simulink model "wang_jingyang_0900085786"  (R2022a)
settings: Solver=FixedStepAuto  StartTime=0.0  StopTime=1  FixedStep=1e-06  MaxStep=1e-6  RelTol=1e-3
values from neighbouring files (symbols this model uses):
  fsw = 1000000    [wang_jingyang_0900085786_parameter.m]
  J = 183e-07    (= 1.83e-05)    [wang_jingyang_0900085786_parameter.m]
  kt = 0.137    [wang_jingyang_0900085786_parameter.m]
  max_current = 2.8    [wang_jingyang_0900085786_parameter.m]
  period_duty = 1    [wang_jingyang_0900085786_parameter.m]
  r = 6.61    [wang_jingyang_0900085786_parameter.m]
  rs = 0.72    [wang_jingyang_0900085786_parameter.m]
  torque_slope = 2.646E-04    (= 0.0002646)    [wang_jingyang_0900085786_parameter.m]
  vs = 72    [wang_jingyang_0900085786_parameter.m]
libraries: nesl_utility x13, ee_lib x10, fl_lib x9, spsMeanLib x2, simulink x2
settings Model: Creator=claudio.rossi  LastModifiedBy=JasonIrayshon
settings SolverCC: ZeroCrossAlgorithm=Adaptive
settings DataIOCC: SaveFormat=Array
settings DebuggingCC: IgnoredZcDiagnostic=none  UnconnectedInputMsg=warning  UnconnectedOutputMsg=warning  UnconnectedLineMsg=warning
settings RTWCC: DLArmComputeVersion=19.05

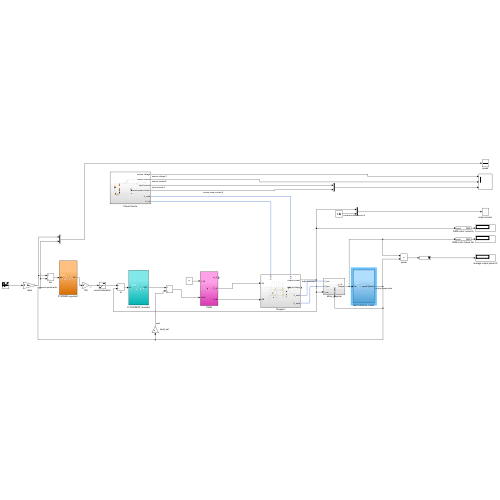
[thumbnail: Simulink's stored preview of the top-level diagram]
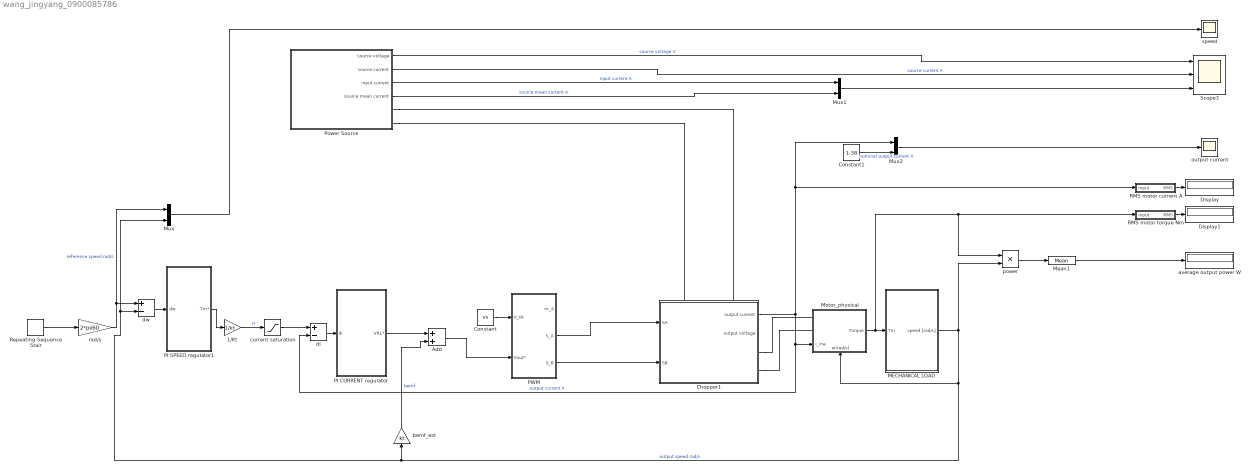
== system wang_jingyang_0900085786 ==
  1/Kt : Gain  Gain=1/kt
  Add : Sum
  Chopper1 : Subsystem
      settings: PortSchema="{\"entries\":[{\"content\":{\"sides\":[{\"content\":{\"connectorIds\":[\"In1\",\"In2\"]},\"type\":\"ConnectorPlacement.EquallySpacedRectSide\",\"uuid\":\"6b8cc3de-865d-4570-879b-f9024d4fd7e5\"},{\"content\":{\"connectorIds\":[\"Out1\",\"Out2\",\"RConn1\",\"RConn2\"],\"side\":\"RIGHT\"},\"type\":\"ConnectorPlacement.EquallySpacedRectSide\",\"uuid\":\"7f03e7c5-24a6-417f-989e-25a3d60ab139\"},{\"content\":{\"connectorIds\":[\"LConn1\",\"LConn2\"],\"side\":\"TOP\"},\"type\":\"ConnectorPlacement.EquallySpacedRectSide\",\"uuid\":\"d8aa3f33-fa7f-4dd9-94c6-a8d4ddf046a0\"},{\"content\":{\"connectorIds\":[],\"side\":\"BOTTOM\"},\"type\":\"ConnectorPlacement.EquallySpacedRectSide\",\"uuid\":\"82a3c5ca-95ba-41a9-9ebb-951a0a94f788\"}]},\"type\":\"ConnectorPlacement.EquallySpacedConnector\",\"uuid\":\"1a04d642-2b5e-450e-b011-8676eb2fa378\"}],\"packageUris\":[\"http://schema.mathworks.com/mf0/Connector/R2020b\"],\"version\":\"1.0\"}"
  Constant : Constant  Value=vs
  Constant1 : Constant  Value=1.38
  Display : Display
  Display1 : Display
  MECHANICAL LOAD : Subsystem
  Mean1 : spsMeanLib/Mean  Freq=fsw  Vinit=0  Ts=0
  Motor_physical : Subsystem
      settings: PortSchema="{\"entries\":[{\"content\":{\"sides\":[{\"content\":{\"connectorIds\":[\"LConn1\",\"LConn2\",\"In1\"]},\"type\":\"ConnectorPlacement.EquallySpacedRectSide\",\"uuid\":\"b6037c4a-1f3a-465c-bacb-bde747a26b4c\"},{\"content\":{\"connectorIds\":[\"Out1\"],\"side\":\"RIGHT\"},\"type\":\"ConnectorPlacement.EquallySpacedRectSide\",\"uuid\":\"519ff893-bc94-47bb-a520-d8eddd14445d\"},{\"content\":{\"connectorIds\":[],\"side\":\"TOP\"},\"type\":\"ConnectorPlacement.EquallySpacedRectSide\",\"uuid\":\"9e95d8c6-7747-4ab4-a157-2e1e9a78c15e\"},{\"content\":{\"connectorIds\":[\"In2\"],\"side\":\"BOTTOM\"},\"type\":\"ConnectorPlacement.EquallySpacedRectSide\",\"uuid\":\"be1431e5-ccb9-4c79-a3a9-fcb6f60af3f0\"}]},\"type\":\"ConnectorPlacement.EquallySpacedConnector\",\"uuid\":\"2d312488-f543-490d-bb4c-a0f0f3bfbb5e\"}],\"packageUris\":[\"http://schema.mathworks.com/mf0/Connector/R2020b\"],\"version\":\"1.0\"}"
  Mux : Mux  Inputs=2
  Mux1 : Mux  Inputs=2
  Mux2 : Mux  Inputs=2
  PI CURRENT regulator : Subsystem
  PI SPEED regulator1 : Subsystem
  PWM : Subsystem
  Power Source : Subsystem
  RMS motor current A : Subsystem  mask{t=period_duty}
      mask prompts: t "Integrating time T [s]"
      mask DialogControl DescTextVar Prompt: Mean value calculator over period T
  RMS motor torque Nm : Subsystem  mask{t=period_duty}
      mask prompts: t "Integrating time T [s]"
      mask DialogControl DescTextVar Prompt: Mean value calculator over period T
  Repeating Sequence Stair : simulink/Sources/Repeating Sequence Stair  OutValues="[0 3375 3375  -1350 675 675 1350 1350 3375 3375].'"  tsamp=0.1  OutMin=[]  OutMax=[]  OutDataTypeStr=double  OutputDataTypeScalingMode=double  OutDataType=fixdt(0,8)  ConRadixGroup=Best Precision: Vector-wise  OutScaling=2^-12
  Scope3 : Scope  NumInputPorts=3
  average output power W : Display
  bemf_est : Gain  Gain=kt
  current saturation : Saturate  UpperLimit=max_current/2  LowerLimit=-max_current/2
  di : Sum  Inputs=+-
  dw : Sum  Inputs=+-
  "output current " : Scope
  power : Product
  rad/s : Gain  Gain=2*pi/60
  speed : Scope
  wires:
  di/1 -> PI CURRENT regulator/1(di)
  bemf_est/1 -> Add/2  "bemf"
  MECHANICAL LOAD/1(speed [rad/s]) -> power/2, Mux/2, dw/2, bemf_est/1, Motor_physical/2(w(rad/s))  "output speed rad/s"
  PI SPEED regulator1/1(Tm*) -> 1/Kt/1
  rad/s/1 -> Mux/1, dw/1  "reference speed rad/s"
  dw/1 -> PI SPEED regulator1/1(dw)
  current saturation/1 -> di/1
  1/Kt/1 -> current saturation/1  "I*"
  RMS motor current A/1(RMS) -> Display/1
  Mux/1 -> speed/1
  PI CURRENT regulator/1(VRL*) -> Add/1
  PWM/2(S_A) -> Chopper1/1(SA)
  PWM/3(S_B) -> Chopper1/2(SB)
  Add/1 -> PWM/2(Vout*)
  RMS motor torque Nm/1(RMS) -> Display1/1
  Chopper1/1(output current) -> RMS motor current A/1(input), Mux2/1, di/2, Motor_physical/1(I_ina)  "output current A"
  Motor_physical/1(Torque) -> RMS motor torque Nm/1(input), power/1, MECHANICAL LOAD/1(Tm)
  Constant/1 -> PWM/1(V_IN)
  Repeating Sequence Stair/1 -> rad/s/1
  Power Source/1(source voltage) -> Scope3/1  "source voltage V"
  Power Source/2(source current) -> Scope3/2  "source current A"
  Power Source/4("source mean current ") -> Mux1/2  "source mean current A"
  Power Source/3(input current) -> Mux1/1  "input current A"
  Mux1/1 -> Scope3/3
  Constant1/1 -> Mux2/2  "nominal output current A"
  Mux2/1 -> "output current "/1
  power/1 -> Mean1/1
  Mean1/1 -> average output power W/1
  connections:
  Power Source/RConn1 -- Chopper1/LConn2
  Power Source/RConn2 -- Chopper1/LConn1
  Chopper1/RConn1 -- Motor_physical/LConn1
  Chopper1/RConn2 -- Motor_physical/LConn2

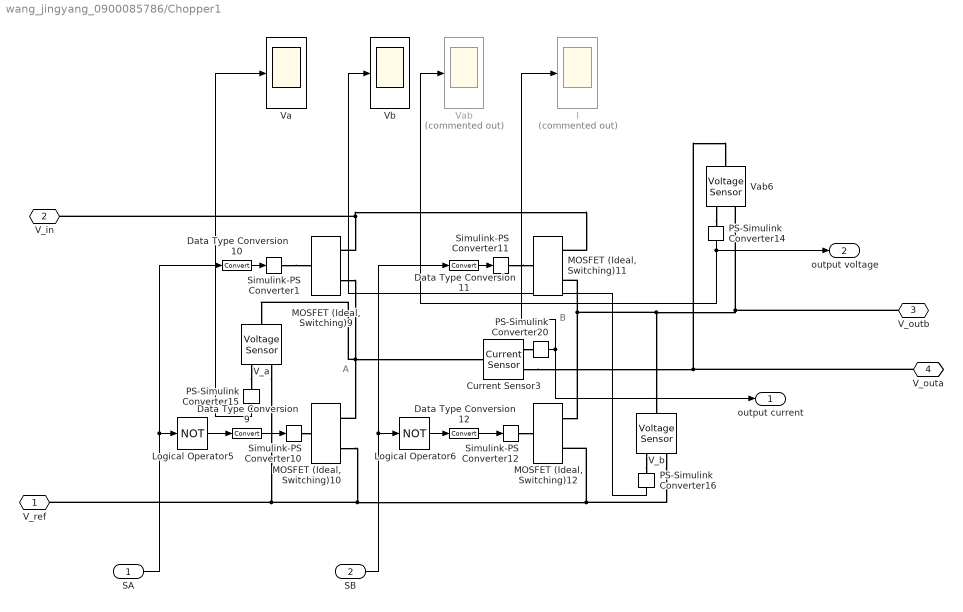
== system wang_jingyang_0900085786/Chopper1 ==
  note: A
  note: B
  SA : Inport
  SB : Inport  Port=2
  Current Sensor3 : fl_lib/Electrical/Electrical Sensors/Current Sensor
      settings: SourceProductBaseCode=PW,SS,VE
  Data Type Conversion{9..12} (4 alike) : DataTypeConversion  SaturateOnIntegerOverflow=off  RndMeth=Floor
  I : Scope  Commented=on
  Logical Operator5 : Logic  Operator=NOT  AllPortsSameDT=off  OutDataTypeStr=boolean
  Logical Operator6 : Logic  Operator=NOT  AllPortsSameDT=off  OutDataTypeStr=boolean
  MOSFET (Ideal, Switching){9..12} (4 alike) : ee_lib/Semiconductors & Converters/MOSFET (Ideal, Switching)  Rds=0.01 Ohm  Goff=1e-6 1/Ohm  Vth=0.5 V  diode_param=1  diode_Vf=0.8 V  diode_Ron=0.001 Ohm  diode_Goff=1e-5 1/Ohm  diode_C=50e-9 F  diode_iRM=-235 A  diode_iF=300 A  diode_idot=-50 A/us  diode_trr_param=1  diode_trr_factor=3  diode_trr=15 us  diode_Qrr=1500 s*uA  thermal_loss_option=ee.enum.converters.thermalLossOption.constantvalues  Von_data=[0, 1.1, 1.3, 1.45, 1.75, 2.25, 2.7; 0, 1, 1.15, 1.35, 1.7, 2.35, 3] V  Tj=[298.15, 398.15] K  Iout_data=[0, 10, 50, 100, 200, 400, 600] A  Eon_data=[0, .29, 1.43, 2.86, 5.71, 13.14, 22.86; 0, .57, 2.63, 5.14, 10.29, 20.57, 30.29] * 1e-3 J  Eoff_data=[0, .21, 1.07, 2.14, 4.29, 9.86, 17.14; 0, .43, 1.97, 3.86, 7.71, 15.43, 22.71] * 1e-3 J  Tj_loss=[298.15, 398.15] K  Iout_data_loss=[0, 10, 50, 100, 200, 400, 600] A  Eon_scalar=22.86e-3 J  Eoff_scalar=17.14e-3 J  Voff=300 V  Iout_scalar=600 A  diodeModelType=ee.enum.converters.diodeModelType.pwl  diodeTableType=ee.enum.diode.tableType.IfMat  diode_IfMat=[.07, .12, .19, 1.75, 4.24, 7.32, 11.2; .16, .3, .72, 2.14, 4.02, 6.35, 9.12] A  diode_VfMat=[.9, 1.15, 1.25, 1.5, 1.75, 2.17, 2.6, 2.85; .58, .68, .75, 1.1, 1.38, 1.77, 2.27, 2.7] V  diode_TjVec=[25, 125] degC  diode_VfVec=[.5, .7, .9, 1.3, 1.7, 2.1, 2.5] V  diode_IfVec=[.1, .2, .5, 1, 2, 4, 7, 10] A  diode_Vr=-600 V  diode_Ls=150 nH  diode_Erec=0.03 J  thermal_network_parameterization=ee.enum.thermalNetworkTopology.external  Rth=[.03, .2] K/W  Rth_Cauer=[.03, .1, .2] K/W  Rth_Foster=[.03, .2] K/W  thermal_mass_parameterization=ee.enum.thermalNetwork.timeconstant  thermal_mass=[3, 25] J/K  thermal_mass_Cauer=[3, 10, 25] J/K  thermal_mass_Foster=[33, 50] J/K  thermal_time_constant=[.1, 5] s  thermal_time_constant_Cauer=[.1, 1, 5] s  thermal_time_constant_Foster=[1, 10] s  thermal_mass_initial_temperatures=[25, 25] degC  thermal_mass_initial_temperatures_Cauer=[25, 25, 25] degC  junction_thermal_mass=0.1 J/K  steadyState_Foster=simscape.enum.onoff.on  Tvec_initial_Foster=[25, 25, 25, 25] degC  no_thermal_network=0  junction_temperature_specify=off  junction_temperature_priority=None  junction_temperature=25 degC  junction_temperature_nominal_specify=off  junction_temperature_nominal_unit=degC  junction_temperature_nominal_value=1  vT_specify=off  vT_priority=None  vT=0 V  vT_nominal_specify=off  vT_nominal_unit=V  vT_nominal_value=1  Qj_specify=off  Qj_priority=None  Qj=0 W  Qj_nominal_specify=off  Qj_nominal_unit=W  Qj_nominal_value=1
  PS-Simulink Converter{14..16,20} (4 alike) : nesl_utility/PS-Simulink Converter  PhysicalDomain=network_engine_domain  SubClassName=ps_output  LeftPortType=input  RightPortType=output  PseudoPeriodic=off  Frequencies=[]  VectorFormat=inherit  Unit=inherit  AffineConversion=off
      settings: SourceProductBaseCode=SS,PW,VE
  Simulink-PS Converter{1,10..12} (4 alike) : nesl_utility/Simulink-PS Converter  PhysicalDomain=network_engine_domain  SubClassName=ps_input  LeftPortType=input  RightPortType=output  PseudoPeriodic=off  Frequencies=[]  NoiseDistribution=none  NoiseParameters=[]  Unit=1  AffineConversion=off  FilteringAndDerivatives=provide  SimscapeFilterOrder=1  InputFilterTimeConstant=0.001  UdotUserProvided=0
      settings: SourceProductBaseCode=SS,PW,VE
  V_a : fl_lib/Electrical/Electrical Sensors/Voltage Sensor
      settings: SourceProductBaseCode=PW,SS,VE
  V_b : fl_lib/Electrical/Electrical Sensors/Voltage Sensor
      settings: SourceProductBaseCode=PW,SS,VE
  Va : Scope
  Vab : Scope  Commented=on
  Vab6 : fl_lib/Electrical/Electrical Sensors/Voltage Sensor
      settings: SourceProductBaseCode=PW,SS,VE
  Vb : Scope
  V_ref : PMIOPort  Side=Left
  V_in : PMIOPort  Port=2  Side=Left
  V_outb : PMIOPort  Port=3  Side=Right
  V_outa : PMIOPort  Port=4  Side=Right
  output current : Outport
  output voltage : Outport  Port=2
  wires:
  Data Type Conversion9/1 -> Simulink-PS Converter10/1
  Logical Operator5/1 -> Data Type Conversion9/1
  SA/1 -> Data Type Conversion10/1, Logical Operator5/1
  PS-Simulink Converter15/1 -> Va/1
  Data Type Conversion11/1 -> Simulink-PS Converter11/1
  PS-Simulink Converter16/1 -> Vb/1
  Data Type Conversion12/1 -> Simulink-PS Converter12/1
  Logical Operator6/1 -> Data Type Conversion12/1
  Data Type Conversion10/1 -> Simulink-PS Converter1/1
  PS-Simulink Converter20/1 -> I/1, output current/1
  PS-Simulink Converter14/1 -> output voltage/1, Vab/1
  SB/1 -> Logical Operator6/1, Data Type Conversion11/1
  connections:
  V_a/RConn1 -- PS-Simulink Converter15/LConn1
  "MOSFET (Ideal, Switching)12"/RConn2 -- "MOSFET (Ideal, Switching)10"/RConn2 -- V_ref/RConn1 -- V_a/RConn2 -- V_b/RConn2
  Current Sensor3/RConn2 -- Vab6/LConn1 -- V_outa/RConn1
  Simulink-PS Converter1/RConn1 -- "MOSFET (Ideal, Switching)9"/LConn1
  V_b/LConn1 -- V_outb/RConn1 -- Vab6/RConn2 -- "MOSFET (Ideal, Switching)11"/RConn2 -- "MOSFET (Ideal, Switching)12"/RConn1
  Current Sensor3/RConn1 -- PS-Simulink Converter20/LConn1
  "MOSFET (Ideal, Switching)10"/RConn1 -- V_a/LConn1 -- Current Sensor3/LConn1 -- "MOSFET (Ideal, Switching)9"/RConn2
  "MOSFET (Ideal, Switching)11"/RConn1 -- V_in/RConn1 -- "MOSFET (Ideal, Switching)9"/RConn1
  Vab6/RConn1 -- PS-Simulink Converter14/LConn1
  Simulink-PS Converter12/RConn1 -- "MOSFET (Ideal, Switching)12"/LConn1
  Simulink-PS Converter10/RConn1 -- "MOSFET (Ideal, Switching)10"/LConn1
  Simulink-PS Converter11/RConn1 -- "MOSFET (Ideal, Switching)11"/LConn1
  V_b/RConn1 -- PS-Simulink Converter16/LConn1

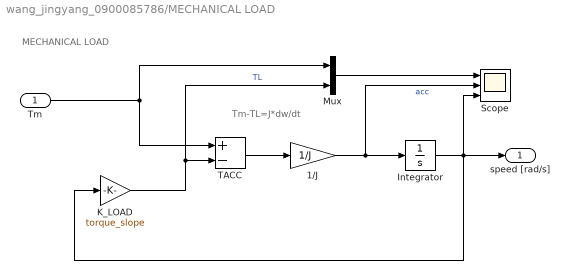
== system wang_jingyang_0900085786/MECHANICAL LOAD ==
  note: MECHANICAL LOAD
  note: Tm-TL=J*dw/dt
  Tm : Inport
  1/J : Gain  Gain=1/J
  Integrator : Integrator
  K_LOAD : Gain  Gain=torque_slope
  Mux : Mux  Inputs=2
  Scope : Scope  NumInputPorts=3
  TACC : Sum  Inputs=+-
  speed [rad/s] : Outport
  wires:
  Tm/1 -> Mux/1, TACC/1
  K_LOAD/1 -> Mux/2, TACC/2  "TL"
  TACC/1 -> 1/J/1
  1/J/1 -> Scope/2, Integrator/1  "acc"
  Integrator/1 -> Scope/3, K_LOAD/1, speed [rad/s]/1
  Mux/1 -> Scope/1

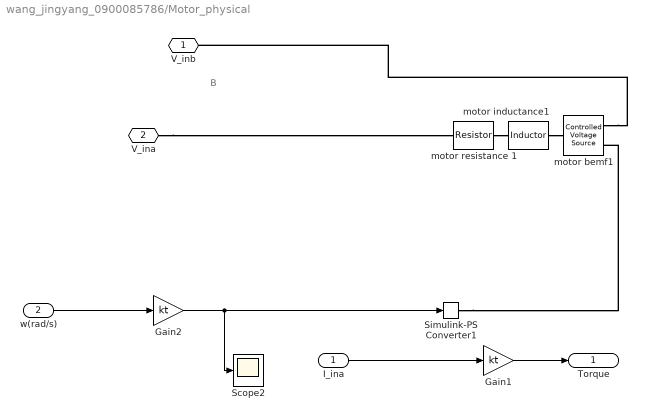
== system wang_jingyang_0900085786/Motor_physical ==
  note: B
  I_ina : Inport
  w(rad/s) : Inport  Port=2
  Gain1 : Gain  Gain=kt
  Gain2 : Gain  Gain=kt
  Scope2 : Scope
  Simulink-PS Converter1 : nesl_utility/Simulink-PS Converter  PhysicalDomain=network_engine_domain  SubClassName=ps_input  LeftPortType=input  RightPortType=output  PseudoPeriodic=off  Frequencies=[]  NoiseDistribution=none  NoiseParameters=[]  Unit=1  AffineConversion=off  FilteringAndDerivatives=provide  SimscapeFilterOrder=1  InputFilterTimeConstant=0.001  UdotUserProvided=0
      settings: SourceProductBaseCode=SS,PW,VE
  motor inductance1 : ee_lib/Passive/Inductor  l=l H  enable_L_tol=0  L_tol=20  tol_distribution=1  nSigma=4  r=0 Ohm  g=1e-9 1/Ohm  enable_operating_limits=0  operating_limit_action=2  max_working_current=1 A  power_rating=1 W  enable_faults=0  fault_action=1  lambdaPercent=50  k_faulted=0.9999  turnsShort=0  openCct=0  groundShort=0  groundShortG=0 1/Ohm  tau_fault=1e-3 s  enable_temporal_fault=0  t_fault=1 s  enable_behavioral_fault=0  max_permissible_voltage=100 V  n_fail_on_voltage=1  max_permissible_current=1 A  t_fail_on_current=1 s  i_L_specify=off  i_L_priority=High  i_L=0 A  i_L_nominal_specify=off  i_L_nominal_unit=A  i_L_nominal_value=1
  motor resistance 1 : ee_lib/Passive/Resistor  R=r Ohm  enable_R_tol=0  R_tol=5  tol_distribution=1  nSigma=4  enable_operating_limits=0  operating_limit_action=2  max_working_voltage=100 V  power_rating=1 W  enable_faults=0  fault_action=1  R_faulted=inf Ohm  enable_temporal_fault=0  t_fault=1 s  enable_behavioral_fault=0  max_permissible_current=1 A  t_fail_on_current=1 s  noise_mode=0  sample_time=1e-3 s  repeatability=1  auto_seed=4144164703  user_seed=0  Tdevice=25 degC  power_derating_T1=70 degC  power_derating_T2=155 degC  operating_temperature_range_vec=[-50, 150] degC  alpha=3.93e-3 1/K  Tmeas=25 degC  thermal_mass=100 J/K  temperature_specify=off  temperature_priority=High  temperature=298.15 K  temperature_nominal_specify=off  temperature_nominal_unit=K  temperature_nominal_value=1
  motor bemf1 : fl_lib/Electrical/Electrical Sources/Controlled Voltage Source
      settings: SourceProductBaseCode=PW,SS,VE
  V_inb : PMIOPort  Side=Left
  V_ina : PMIOPort  Port=2  Side=Left
  Torque : Outport
  wires:
  I_ina/1 -> Gain1/1
  Gain2/1 -> Scope2/1, Simulink-PS Converter1/1
  Gain1/1 -> Torque/1
  w(rad/s)/1 -> Gain2/1
  connections:
  motor resistance 1/RConn1 -- motor inductance1/LConn1
  motor bemf1/RConn2 -- V_inb/RConn1
  V_ina/RConn1 -- motor resistance 1/LConn1
  Simulink-PS Converter1/RConn1 -- motor bemf1/RConn1
  motor inductance1/RConn1 -- motor bemf1/LConn1

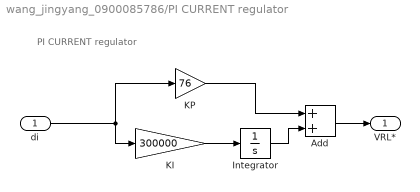
== system wang_jingyang_0900085786/PI CURRENT regulator ==
  note: PI CURRENT regulator
  di : Inport
  Add : Sum
  Integrator : Integrator
  KI : Gain  Gain=300000
  KP : Gain  Gain=76
  VRL* : Outport
  wires:
  Integrator/1 -> Add/2
  di/1 -> KP/1, KI/1
  KP/1 -> Add/1
  KI/1 -> Integrator/1
  Add/1 -> VRL*/1

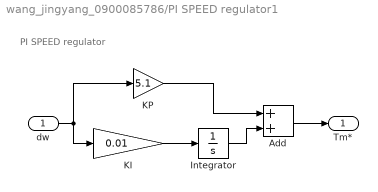
== system wang_jingyang_0900085786/PI SPEED regulator1 ==
  note: PI SPEED regulator
  dw : Inport
  Add : Sum
  Integrator : Integrator
  KI : Gain  Gain=0.01
  KP : Gain  Gain=5.1
  Tm* : Outport
  wires:
  Add/1 -> Tm*/1
  KI/1 -> Integrator/1
  KP/1 -> Add/1
  dw/1 -> KI/1, KP/1
  Integrator/1 -> Add/2

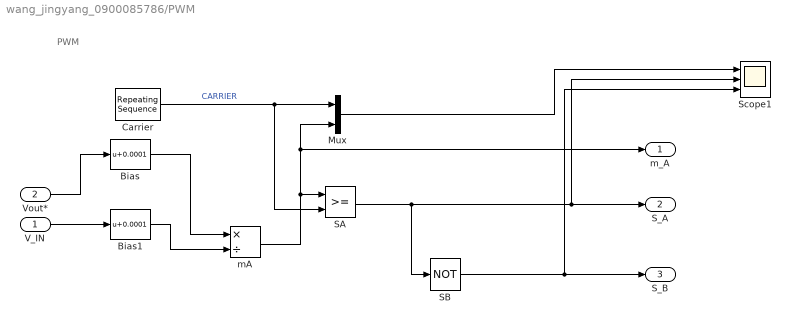
== system wang_jingyang_0900085786/PWM ==
  note: PWM
  V_IN : Inport
  Vout* : Inport  Port=2
  Bias : Bias  Bias=0.0001  SaturateOnIntegerOverflow=off
  Bias1 : Bias  Bias=0.0001  SaturateOnIntegerOverflow=off
  Carrier : simulink/Sources/Repeating Sequence  rep_seq_t="[0 1/fsw/2  1/fsw]"  rep_seq_y=[-1 1 -1]
  Mux : Mux  Inputs=2
  SA : RelationalOperator  OutDataTypeStr=boolean  RndMeth=Simplest  InputSameDT=off
  SB : Logic  Operator=NOT  AllPortsSameDT=off  OutDataTypeStr=boolean
  Scope1 : Scope  NumInputPorts=3
  mA : Product  Inputs=*/
  m_A : Outport
  S_A : Outport  Port=2
  S_B : Outport  Port=3
  wires:
  Carrier/1 -> SA/2, Mux/1  "CARRIER"
  SA/1 -> SB/1, Scope1/2, S_A/1
  Mux/1 -> Scope1/1
  mA/1 -> Mux/2, m_A/1, SA/1
  SB/1 -> Scope1/3, S_B/1
  Vout*/1 -> Bias/1
  Bias/1 -> mA/1
  V_IN/1 -> Bias1/1
  Bias1/1 -> mA/2

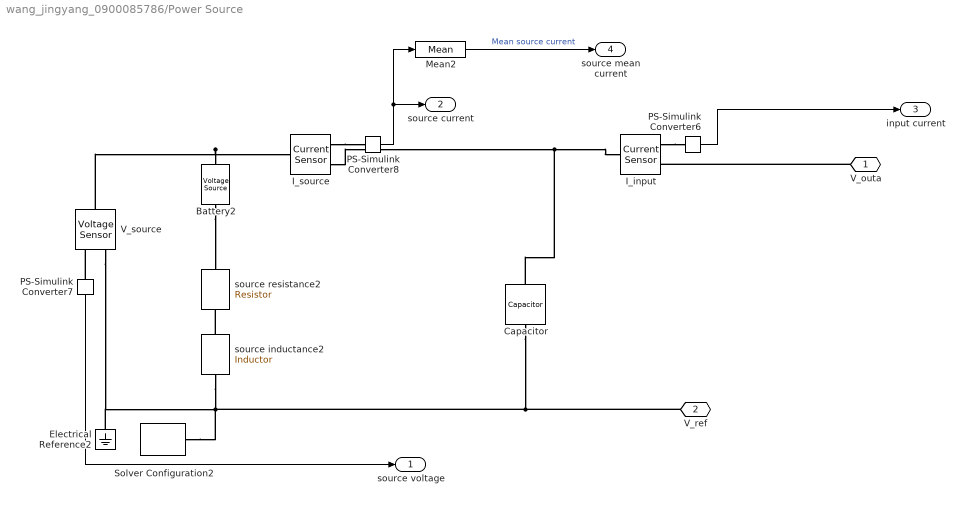
== system wang_jingyang_0900085786/Power Source ==
  Battery2 : ee_lib/Sources/Voltage Source  dc_voltage=vs V  ac_voltage=0 V  ac_shift=0 rad  ac_frequency=60 Hz  noise_mode=0  PSD=0 V^2/Hz  repeatability=1  auto_seed=676943032  user_seed=0  sample_time=1e-3 s  i_specify=off  i_priority=None  i=0 A  i_nominal_specify=off  i_nominal_unit=A  i_nominal_value=1  v_specify=off  v_priority=None  v=0 V  v_nominal_specify=off  v_nominal_unit=V  v_nominal_value=1
  Capacitor : ee_lib/Passive/Capacitor  cap_option=0  c=940e-5 F  Cvec=[1e-05, 1e-06] F  Vvec=[0, 10] V  CV_table_symmetry=1  f_vec=[1, 10] kHz  DFext_vec=[.8, 1.2]  enable_C_tol=0  C_tol=5  tol_distribution=1  nSigma=4  r=0.21 Ohm  g=0 1/Ohm  averaging_period=0 s  enable_operating_limits=0  operating_limit_action=2  max_working_voltage_range=[-25, 25] V  power_rating=1 W  enable_faults=0  fault_action=1  Cscale_faulted=100  R_faulted=1e-3 Ohm  G_faulted=0 1/Ohm  tau_fault=1e-3 s  enable_temporal_fault=0  t_fault=1 s  enable_behavioral_fault=0  max_permissible_voltage_range=[-100, 100] V  t_fail_on_voltage=1 s  i_specify=off  i_priority=None  i=0 A  i_nominal_specify=off  i_nominal_unit=A  i_nominal_value=1  v_specify=off  v_priority=None  v=0 V  v_nominal_specify=off  v_nominal_unit=V  v_nominal_value=1  vc_specify=off  vc_priority=High  vc=0 V  vc_nominal_specify=off  vc_nominal_unit=V  vc_nominal_value=1
  Electrical Reference2 : fl_lib/Electrical/Electrical Elements/Electrical Reference
      settings: SourceProductBaseCode=PW,SS,VE
  I_input : fl_lib/Electrical/Electrical Sensors/Current Sensor
      settings: SourceProductBaseCode=PW,SS,VE
  I_source : fl_lib/Electrical/Electrical Sensors/Current Sensor
      settings: SourceProductBaseCode=PW,SS,VE
  Mean2 : spsMeanLib/Mean  Freq=fsw  Vinit=0  Ts=0
  PS-Simulink Converter6 : nesl_utility/PS-Simulink Converter  PhysicalDomain=network_engine_domain  SubClassName=ps_output  LeftPortType=input  RightPortType=output  PseudoPeriodic=off  Frequencies=[]  VectorFormat=inherit  Unit=inherit  AffineConversion=off
      settings: SourceProductBaseCode=SS,PW,VE
  PS-Simulink Converter7 : nesl_utility/PS-Simulink Converter  PhysicalDomain=network_engine_domain  SubClassName=ps_output  LeftPortType=input  RightPortType=output  PseudoPeriodic=off  Frequencies=[]  VectorFormat=inherit  Unit=inherit  AffineConversion=off
      settings: SourceProductBaseCode=SS,PW,VE
  PS-Simulink Converter8 : nesl_utility/PS-Simulink Converter  PhysicalDomain=network_engine_domain  SubClassName=ps_output  LeftPortType=input  RightPortType=output  PseudoPeriodic=off  Frequencies=[]  VectorFormat=1-D array  Unit=inherit  AffineConversion=off
      settings: SourceProductBaseCode=SS,PW,VE
  Solver Configuration2 : nesl_utility/Solver Configuration  PhysicalDomain=network_engine_domain  SubClassName=solver  LeftPortType=input  RightPortType=generic  Tones=[]  Harmonics=[]  SimulateNoise=off  Profile=off  UseLocalSampling=off  EnableSwitchedLinearOptims=on  FrequencyDomain=off  UseCCode=off  RelTol=0.001  AbsTol=1e-06  MinStep=1e-09  ToWorkspace=off  RevertToSquareIcSolve=off  NumHomotopyIterations=100  PhasorMode=off  PhasorModeNumHarmonics=1  IndexReductionMethod=DerivativeReplacement  DoDC=off  ResidualTolerance=1e-09  UseLocalSolver=off  LocalSolverChoice=NE_BACKWARD_EULER_ADVANCER  LocalSolverSampleTime=0.001  DoFixedCost=off  MaxNonlinIter=3  MaxModeIter=2  ComputeImpulses=off  ImpulseIterations=2  LinearAlgebra=auto  LinearAlgebraNumThread=0  EquationFormulation=NE_TIME_EF  DelaysMemoryBudget=1024  AutomaticFiltering=on  FilteringTimeConstant=0.001  PartitionStorageMethod=AS_NEEDED  PartitionMemoryBudget=1024  PartitionMethod=ROBUST
      settings: SourceProductBaseCode=SS,PW,VE
  V_source : fl_lib/Electrical/Electrical Sensors/Voltage Sensor
      settings: SourceProductBaseCode=PW,SS,VE
  source inductance2 : ee_lib/Passive/Inductor  l=ls mH  enable_L_tol=0  L_tol=20  tol_distribution=1  nSigma=4  r=0 Ohm  g=1e-9 1/Ohm  enable_operating_limits=0  operating_limit_action=2  max_working_current=1 A  power_rating=1 W  enable_faults=0  fault_action=1  lambdaPercent=50  k_faulted=0.9999  turnsShort=0  openCct=0  groundShort=0  groundShortG=0 1/Ohm  tau_fault=1e-3 s  enable_temporal_fault=0  t_fault=1 s  enable_behavioral_fault=0  max_permissible_voltage=100 V  n_fail_on_voltage=1  max_permissible_current=1 A  t_fail_on_current=1 s  i_L_specify=off  i_L_priority=High  i_L=0 A  i_L_nominal_specify=off  i_L_nominal_unit=A  i_L_nominal_value=1
  source resistance2 : ee_lib/Passive/Resistor  R=rs Ohm  enable_R_tol=0  R_tol=5  tol_distribution=1  nSigma=4  enable_operating_limits=0  operating_limit_action=2  max_working_voltage=100 V  power_rating=1 W  enable_faults=0  fault_action=1  R_faulted=inf Ohm  enable_temporal_fault=0  t_fault=1 s  enable_behavioral_fault=0  max_permissible_current=1 A  t_fail_on_current=1 s  noise_mode=0  sample_time=1e-3 s  repeatability=1  auto_seed=4168664255  user_seed=0  Tdevice=25 degC  power_derating_T1=70 degC  power_derating_T2=155 degC  operating_temperature_range_vec=[-50, 150] degC  alpha=3.93e-3 1/K  Tmeas=25 degC  thermal_mass=100 J/K  temperature_specify=off  temperature_priority=High  temperature=298.15 K  temperature_nominal_specify=off  temperature_nominal_unit=K  temperature_nominal_value=1
  V_outa : PMIOPort  Side=Right
  V_ref : PMIOPort  Port=2  Side=Right
  source voltage : Outport
  source current : Outport  Port=2
  input current : Outport  Port=3
  "source mean current " : Outport  Port=4
  wires:
  PS-Simulink Converter8/1 -> Mean2/1, source current/1
  PS-Simulink Converter7/1 -> source voltage/1
  PS-Simulink Converter6/1 -> input current/1
  Mean2/1 -> "source mean current "/1  "Mean source current"
  connections:
  PS-Simulink Converter7/LConn1 -- V_source/RConn1
  I_source/RConn2 -- I_input/LConn1 -- Capacitor/LConn1
  I_input/RConn1 -- PS-Simulink Converter6/LConn1
  I_source/RConn1 -- PS-Simulink Converter8/LConn1
  source inductance2/LConn1 -- source resistance2/RConn1
  Battery2/LConn1 -- I_source/LConn1 -- V_source/LConn1
  V_ref/RConn1 -- Solver Configuration2/RConn1 -- source inductance2/RConn1 -- V_source/RConn2 -- Electrical Reference2/LConn1 -- Capacitor/RConn1
  V_outa/RConn1 -- I_input/RConn2
  Battery2/RConn1 -- source resistance2/LConn1

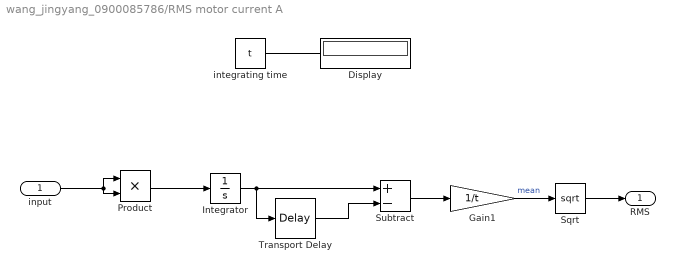
== system wang_jingyang_0900085786/RMS motor current A ==
  input : Inport
  Display : Display
      settings: Format=short_e  Floating=on
  Gain1 : Gain  Gain=1/t
  Integrator : Integrator
  Product : Product
  Sqrt : Sqrt
  Subtract : Sum  Inputs=+-
  Transport Delay : TransportDelay  DelayTime=t
  integrating time : Constant  Value=t
  RMS : Outport
  wires:
  integrating time/1 -> ?
  Transport Delay/1 -> Subtract/2
  Integrator/1 -> Transport Delay/1, Subtract/1
  Subtract/1 -> Gain1/1
  input/1 -> Product/1, Product/2
  Product/1 -> Integrator/1
  Sqrt/1 -> RMS/1
  Gain1/1 -> Sqrt/1  "mean"

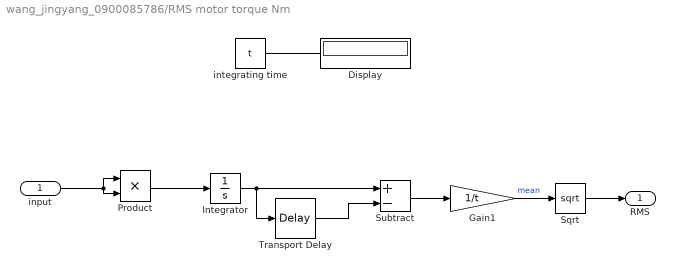
== system wang_jingyang_0900085786/RMS motor torque Nm ==
  input : Inport
  Display : Display
      settings: Format=short_e  Floating=on
  Gain1 : Gain  Gain=1/t
  Integrator : Integrator
  Product : Product
  Sqrt : Sqrt
  Subtract : Sum  Inputs=+-
  Transport Delay : TransportDelay  DelayTime=t
  integrating time : Constant  Value=t
  RMS : Outport
  wires:
  integrating time/1 -> ?
  Transport Delay/1 -> Subtract/2
  Integrator/1 -> Transport Delay/1, Subtract/1
  Subtract/1 -> Gain1/1
  input/1 -> Product/1, Product/2
  Product/1 -> Integrator/1
  Sqrt/1 -> RMS/1
  Gain1/1 -> Sqrt/1  "mean"
